simulink subsystem "PIDControllerSub"  (R2024b)
settings: Solver=VariableStepAuto  StartTime=0.0  StopTime=10.0  RelTol=1e-3
undefined symbols (not defined in the file): k, ki, Ts
settings Model: Creator=flyingtopher  LastModifiedBy=flyingtopher

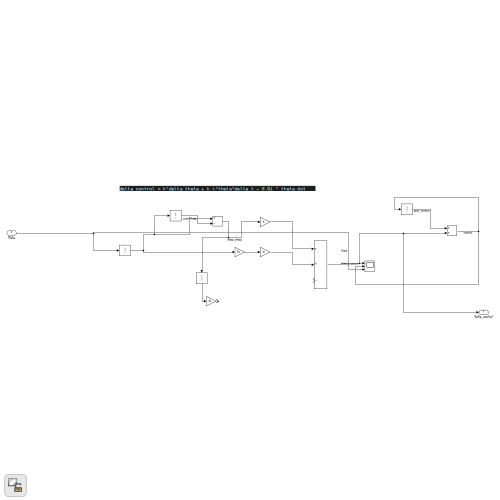
[thumbnail: Simulink's stored preview of the top-level diagram]
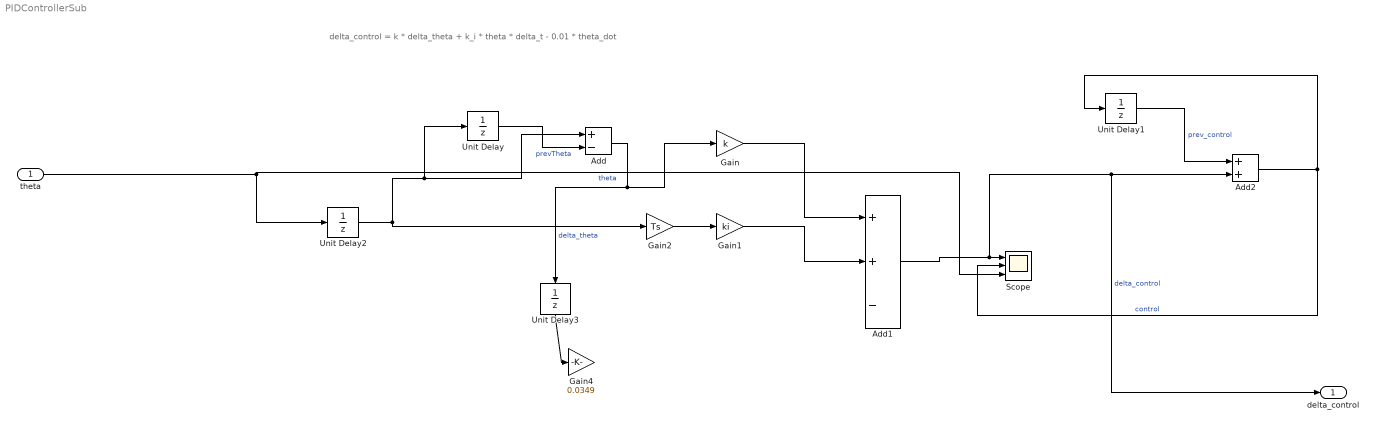
== system PIDControllerSub ==
  note: delta_control = k * delta_theta + k_i * theta * delta_t - 0.01 * theta_dot
  theta : Inport
  Add : Sum  Inputs=+-
  Add1 : Sum  Inputs=++-
  Add2 : Sum
  Gain : Gain  Gain=k
  Gain1 : Gain  Gain=ki
  Gain2 : Gain  Gain=Ts
  Gain4 : Gain  Gain=0.0349
  Scope : Scope  NumInputPorts=3
  Unit Delay : UnitDelay  InitialCondition=1  SampleTime=Ts  HasFrameUpgradeWarning=on
  Unit Delay1 : UnitDelay  InitialCondition=2  SampleTime=-1  HasFrameUpgradeWarning=on
  Unit Delay2 : UnitDelay  SampleTime=-1  HasFrameUpgradeWarning=on
  Unit Delay3 : UnitDelay  SampleTime=-1  HasFrameUpgradeWarning=on
  delta_control : Outport
  wires:
  Add/1 -> Gain/1, Unit Delay3/1  "delta_theta"
  Gain1/1 -> Add1/2
  Gain2/1 -> Gain1/1
  theta/1 -> Scope/3, Unit Delay2/1  "theta"
  Gain/1 -> Add1/1
  Unit Delay1/1 -> Add2/1  "prev_control"
  Unit Delay/1 -> Add/2  "prevTheta"
  Add2/1 -> Scope/2, Unit Delay1/1  "control"
  Add1/1 -> Scope/1, Add2/2, delta_control/1  "delta_control"
  Unit Delay2/1 -> Add/1, Unit Delay/1, Gain2/1
  Unit Delay3/1 -> Gain4/1
